simulink model "sens_example_PID_sim"  (R2017a)
settings: Solver=ode5  StartTime=0.0  StopTime=10.0  FixedStep=0.25  MaxStep=0.01  RelTol=1e-3  EnableMultiTasking=on
model workspace (MAT data in the model file):
  a1 = 2
  a2 = 4
  b2 = 3.2
  p = [2.65723736536; 1.93381365527; 3.98280422144]
libraries: simulink_extras x1
settings Model: ExtModeTrigMode=oneshot  ExtModeArmWhenConnect=off  Creator=CarlosMario  LastModifiedBy=drojasd
settings SolverCC: AutoInsertRateTranBlk=on  InsertRTBMode=Never (minimum delay)
settings DataIOCC: SaveFormat=Array  SignalLoggingSaveFormat=ModelDataLogs  SignalLogging=off  DSMLogging=off  ReturnWorkspaceOutputs=on  OutputTimes=tout
settings OptimizationCC: BlockReduction=off  BooleanDataType=off  LifeSpan=inf
settings DebuggingCC: SaveWithParameterizedLinksMsg=none  UnderspecifiedInitializationDetection=Classic  MergeDetectMultiDrivingBlocksExec=none  SignalResolutionControl=TryResolveAllWithWarning  MultiTaskDSMMsg=warning  MultiTaskCondExecSysMsg=none  StateNameClashWarn=warning  SFUnexpectedBacktrackingDiag=warning  SFNoUnconditionalDefaultTransitionDiag=warning  SFExecutionAtInitializationDiag=none
settings HardwareCC: ProdBitPerPointer=32  ProdBitPerSizeT=32  ProdBitPerPtrDiffT=32  ProdLargestAtomicFloat=None  ProdIntDivRoundTo=Undefined  ProdEndianess=Unspecified  ProdWordSize=32  ProdHWDeviceType=32-bit Generic  TargetUnknown=on
settings ModelReferenceCC: PropagateSignalLabelsOutOfModel=off
settings GRTTargetCC: TargetLangStandard=C89/C90 (ANSI)  GeneratePreprocessorConditionals=Disable all  CombineOutputUpdateFcns=off  GRTInterface=on
settings ConfigComp: CovMetricSettings=dw  CovHtmlReporting=on  CovSaveCumulativeToWorkspaceVar=on  CovSaveSingleToWorkspaceVar=on  CovExternalEMLEnable=off

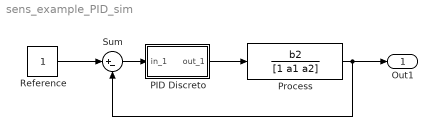
== system sens_example_PID_sim ==
  PID Discreto : Subsystem  mask(Discrete PID Control){kp=3.34, Ti=0.73, Td=0.17, u=[-100 100], ini=0, T=0.25}
      mask prompts: u "Control input range [umin, umax]"; ini "Initial control input"; T "Sample time (Ts)"
      mask help: u(k) = Kp*[ e(k) + (1/Ti)*int(e) + Td*e' ]
      mask init:
      | umin=u(1); umax=u(2);
      mask Display:
      | disp('Discrete\nPID')
      | port_label('input',1,'e')
      | port_label('output',1,'u')
  Process : TransferFcn  Numerator=b2  Denominator=[1 a1 a2]
  Reference : Constant
  Sum : Sum  Inputs=|+-  SaturateOnIntegerOverflow=on  InputSameDT=on  OutDataTypeStr=Inherit: Same as first input
  Out1 : Outport
  wires:
  Reference/1 -> Sum/1
  Sum/1 -> PID Discreto/1(in_1)
  PID Discreto/1(out_1) -> Process/1
  Process/1 -> Out1/1, Sum/2

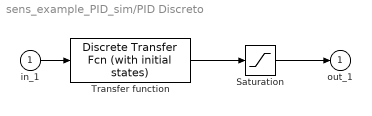
== system sens_example_PID_sim/PID Discreto ==
  in_1 : Inport
  Saturation : Saturate  UpperLimit=umax  LowerLimit=umin
  Transfer function : simulink_extras/Additional Discrete/Discrete Transfer Fcn (with initial states)  N=[kp*(1+T/(2*Ti)+Td/T) -kp*(1+2*Td/T-T/(2*Ti)) kp*Td/T]  D=[1 -1 0]  X0=ini  TS=T
      settings: SourceProductName=Simulink  SourceProductBaseCode=SL
  out_1 : Outport  InitialOutput=0
  wires:
  Saturation/1 -> out_1/1
  in_1/1 -> Transfer function/1
  Transfer function/1 -> Saturation/1
